simulink model "URController"  (R2023a)
settings: Solver=ode4  StartTime=0.0  StopTime=3  FixedStep=0.001  RelTol=1e-3  EnableMultiTasking=on
values from neighbouring files (symbols this model uses):
  CYCLE_FREQ = 0.001    [init.m]
  MAX_ACC = 100    [init.m]
  MAX_VEL = 180    [init.m]
libraries: slpidlib x13, forwardkinematics x2, simulink x1
(part 3 of 3)

== matlab function URController/Subsystem/Control System/motionGenerator1/MATLAB Function ==
  settings: updateMethod=DISCRETE
  data: posRef input; pos input; vel input; tB output; maxAcc input; maxVel input; dB output; tA output; dA output; dCV output; tCV output; s output; vT output; tD output; sM output; t output; CYCLE_FREQ input; oP output; oV output
% oldPose: initial 0 and loop with output pos
% oldvel: initial 0 and loop with output vel

function [tB, dB, tA, dA, dCV, tCV, s, vT, tD, sM, t, oP, oV] = motionGenerator(posRef, pos, vel, maxAcc, maxVel, CYCLE_FREQ)
    persistent timeBrake distanceBrake;
    persistent timeAccelerate distanceAccelerate;
    persistent distanceConstVelocity timeConstVelocity;
    persistent timeDecelerate;
    persistent shape velTop signM;
    persistent oldPoseRef oldPos oldVel;
    persistent time;
    
    % Initialize the first time the function is called
    if (isempty(timeBrake) || isempty(distanceBrake) || isempty(timeAccelerate) || isempty(distanceAccelerate) ...
            || isempty(distanceConstVelocity) || isempty(timeConstVelocity) || isempty(timeDecelerate) ...
            || isempty(shape) || isempty(velTop) || isempty(signM) || isempty(oldPoseRef) || isempty(oldPos) ...
            || isempty(oldVel) || isempty(time))
        timeBrake = 0;
        distanceBrake = 0;
        timeAccelerate = 0;
        distanceAccelerate = 0;
        distanceConstVelocity = 0;
        timeConstVelocity = 0;
        timeDecelerate = 0;
        shape = 0;
        velTop = 0;
        signM = 0;
        oldPoseRef = 0;
        oldPos = 0;
        oldVel = 0;
        time = 0;

        tB = timeBrake;
        dB = distanceBrake;
        tA = timeAccelerate;
        dA = distanceAccelerate;
        dCV = distanceConstVelocity;
        tCV = timeConstVelocity;
        tD = timeDecelerate;
        s = shape;
        vT = velTop;
        sM = signM;
        t = time;
        oV = oldVel;
        oP = oldPos;
        return;
    end
    
    if (oldPoseRef ~= posRef)
        oldPos = pos;
        oldVel = vel;
        oldPoseRef = posRef;
        time = 0;

        tB = abs(oldVel) / maxAcc;
        dB = tB * abs(oldVel) / 2;
    
        sM = sign(posRef - (oldPos + sign(oldVel)*dB));
        
        if (sM ~= sign(oldVel))  % means brake is needed
            tA = (maxVel / maxAcc);
            dA = tA * (maxVel / 2);
        else
            tB = 0;
            dB = 0;
            tA = (maxVel - abs(oldVel)) / maxAcc;
            dA = tA * (maxVel + abs(oldVel)) / 2;
        end
    
        distanceTotal = abs(posRef - oldPos + sM*dB);
                    
        tD = maxVel / maxAcc;
        distanceDecelerate = tD * (maxVel) / 2;
        dCV = distanceTotal - (dA + distanceDecelerate);
        tCV = dCV / maxVel;
    
        if (tCV > 0)    % trapezoidal s
            s = 1;
            vT = 0;
        else                % triangular s
            s = 0;
            % Recalculate distances and periods
            if (sM ~= sign(oldVel))  % means brake is needed
                vT = sqrt(maxAcc*(distanceTotal));
                tA = (vT / maxAcc);
                dA = tA * (vT / 2);
            else
                tB = 0;
                dB = 0;
                distanceTotal = abs(posRef - oldPos);      % recalculate total distance
                vT = sqrt(0.5*oldVel^2 + maxAcc*distanceTotal);
                tA = (vT - abs(oldVel)) / maxAcc;
                dA = tA * (vT + abs(oldVel)) / 2;
            end
            tD = vT / maxAcc;
            distanceDecelerate = tD * (vT) / 2;
        end
        timeBrake = tB;
        distanceBrake = dB;
        timeAccelerate = tA;
        distanceAccelerate = dA;
        distanceConstVelocity = dCV;
        timeConstVelocity = tCV;
        timeDecelerate = tD;
        shape = s;
        velTop = vT;
        signM = sM;
        oV = oldVel;
        oP = oldPos;
    end
    
    tB = timeBrake;
    dB = distanceBrake;
    tA = timeAccelerate;
    dA = distanceAccelerate;
    dCV = distanceConstVelocity;
    tCV = timeConstVelocity;
    tD = timeDecelerate;
    s = shape;
    vT = velTop;
    sM = signM;
    time = time + CYCLE_FREQ;
    t = time;
    oV = oldVel;
    oP = oldPos;
end

== matlab function URController/Subsystem/Control System/motionGenerator1/MATLAB Function1 ==
  data: timeBrake input; distanceBrake input; timeAccelerate input; distanceAccelerate input; distanceConstVelocity input; timeConstVelocity input; shape input; velTop input; timeDecelerate input; signM input; deltaTime input; posRef input; pos output; vel output; oldPos input; oldVel input; maxAcc input; maxVel input; acc output
function [pos, vel, acc]   = calculateTrapezoidalProfile(timeBrake, distanceBrake, timeAccelerate, ...
    distanceAccelerate, distanceConstVelocity, timeConstVelocity, shape,  velTop, timeDecelerate, ...
    signM, deltaTime, posRef, oldPos, oldVel, maxAcc, maxVel)
    
    t = deltaTime;
    acc = 0;
    
    if (shape)   % trapezoidal shape
        if (t <= (timeBrake+timeAccelerate))
            pos = oldPos + oldVel*t + signM * 0.5*maxAcc*t^2;
            vel = oldVel + signM * maxAcc*t;
            acc = signM * maxAcc;
        elseif (t > (timeBrake+timeAccelerate) && t < (timeBrake+timeAccelerate+timeConstVelocity))
            pos = oldPos + signM * (-distanceBrake + distanceAccelerate + maxVel*(t-timeBrake-timeAccelerate));
            vel = signM * maxVel;
            % MG.acc = 0;
        elseif (t >= (timeBrake+timeAccelerate+timeConstVelocity) && t < (timeBrake+timeAccelerate+timeConstVelocity+timeDecelerate))
            pos = oldPos + signM * (-distanceBrake + distanceAccelerate + distanceConstVelocity + maxVel*(t-timeBrake-timeAccelerate-timeConstVelocity) - 0.5*maxAcc*(t-timeBrake-timeAccelerate-timeConstVelocity)^2);
            vel = signM * (maxVel - maxAcc*(t-timeBrake-timeAccelerate-timeConstVelocity));
            acc = - signM * maxAcc;
        else
            pos = posRef;
            vel = 0;
            % MG.acc = 0;
        end
    else            % triangular shape
        if (t <= (timeBrake+timeAccelerate))
            pos = oldPos + oldVel*t + signM * 0.5*maxAcc*t^2;
            vel = oldVel + signM * maxAcc*t;
            acc = signM * maxAcc;
        elseif (t > (timeBrake+timeAccelerate) && t < (timeBrake+timeAccelerate+timeDecelerate))
            pos = oldPos + signM * (-distanceBrake + distanceAccelerate + velTop*(t-timeBrake-timeAccelerate) - 0.5*maxAcc*(t-timeBrake-timeAccelerate)^2);
            vel = signM * (velTop - maxAcc*(t-timeBrake-timeAccelerate));
            acc = - signM * maxAcc;
        else
            pos = posRef;
            vel = 0;
            acc = 0;
        end
        
    end

end
